simulink model "Consensus_ARdrone"  (R2017b)
settings: Solver=VariableStepAuto  StartTime=0.0  StopTime=100  MinStep=0.001  RelTol=1e-3
values from neighbouring files (symbols this model uses):
  A = zeros(n,n)    [Initial.m]    (also in matlab_promjena_form.mat = [0 1 1 1 1 1 0 1 1 1 1 1 ... (25 elements, 5x5)])
  c_d = 2.5    [Initial.m]    (also in ardrone_params.m; matlab_promjena_form.mat)
  G = zeros(n,n)    [Initial.m]    (also in matlab_promjena_form.mat = [0 0.05 0.05 0.05 0.05 0.05 0 0.05 0.05 0.05 0.05 0.05 ... ()
  g = 9.81    [Initial.m]    (also in ardrone_params.m; matlab_promjena_form.mat)
  Krug = [6.12323399574e-16 0 0 0 0 0 0 5.61829545926e-10 1.42391980871e-11 2.79677204721e-07 7.08910845246e-09 0.000111130804722 ... (72051 elements, 7x10293)]    [Krug.mat]
  m = 1.65    [Initial.m]    (also in ardrone_params.m; matlab_promjena_form.mat)
  pitch_max = 0.4    [Initial.m]    (also in ardrone_params.m; matlab_promjena_form.mat)
  R1 = [0, -1, -1, -2, -2; 0, 1,-1, 2, -2]    [Initial.m]    (also in matlab_promjena_form.mat = [0  -1  -1  -2  -2; 0  1  -1  2  -2])
  R2 = [9, 7, 5 ,3, 1; 0,0,0,0,0]    [Initial.m]    (also in matlab_promjena_form.mat = [9  7  5  3  1; 0  0  0  0  0])
  roll_max = 0.4    [Initial.m]    (also in ardrone_params.m; matlab_promjena_form.mat)
  T_pitch = 0.4    [Initial.m]    (also in ardrone_params.m; matlab_promjena_form.mat)
  T_roll = 0.4    [Initial.m]    (also in ardrone_params.m; matlab_promjena_form.mat)
  T_yaw = 0.8    [Initial.m]    (also in ardrone_params.m; matlab_promjena_form.mat)
  T_z = 0.6    [Initial.m]    (also in ardrone_params.m; matlab_promjena_form.mat)
  x0 = [20, -10, -20, 10, -20]    [Initial.m]    (also in matlab_promjena_form.mat = [0 -1 -1 -2 -2])
  y0 = [20, 10,0, -10, -20]    [Initial.m]    (also in matlab_promjena_form.mat = [0 1 -1 2 -2])
  yaw_rate_max = 0.7864    [Initial.m]    (also in ardrone_params.m; matlab_promjena_form.mat)
  z_rate_max = 0.7    [Initial.m]    (also in ardrone_params.m; matlab_promjena_form.mat)
settings Model: Creator=Mare  LastModifiedBy=Mare

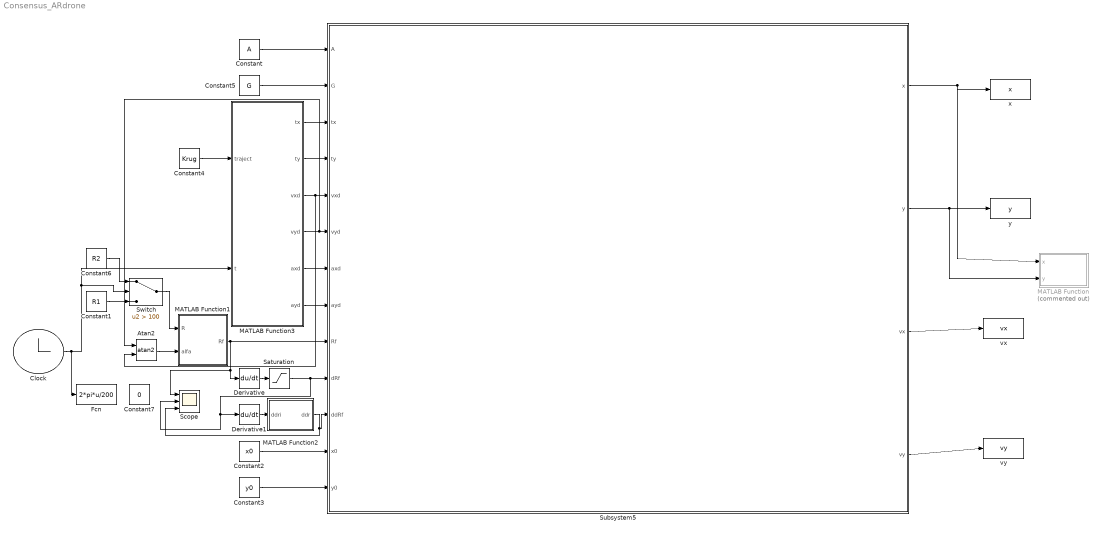
== system Consensus_ARdrone ==
  Atan2 : Trigonometry  Operator=atan2
  Clock : Clock
  Constant : Constant  Value=A
  Constant1 : Constant  Value=R1
  Constant2 : Constant  Value=x0
  Constant3 : Constant  Value=y0
  Constant4 : Constant  Value=Krug
  Constant5 : Constant  Value=G
  Constant6 : Constant  Value=R2
  Constant7 : Constant  Value=0
  Derivative : Derivative
  Derivative1 : Derivative
  Fcn : Fcn  Expr=2*pi*u/200
  MATLAB Function : MATLAB Function  Commented=on  TreatAsAtomicUnit=on
  MATLAB Function1 : MATLAB Function  TreatAsAtomicUnit=on
  MATLAB Function2 : MATLAB Function  TreatAsAtomicUnit=on
  MATLAB Function3 : MATLAB Function  TreatAsAtomicUnit=on
  Saturation : Saturate  UpperLimit=2.5  LowerLimit=-2.5
  Scope : Scope  NumInputPorts=3
  Subsystem5 : Subsystem
  Switch : Switch  Criteria=u2 > Threshold  Threshold=100
  vx : ToWorkspace  VariableName=vx  SaveFormat=Structure With Time  SampleTime=0.5
  vy : ToWorkspace  VariableName=vy  SaveFormat=Structure With Time  SampleTime=0.5
  x : ToWorkspace  VariableName=x  SaveFormat=Structure With Time  SampleTime=0.5
  y : ToWorkspace  VariableName=y  SaveFormat=Structure With Time  SampleTime=0.5
  wires:
  Constant/1 -> Subsystem5/1(A)
  MATLAB Function1/1(Rf) -> Subsystem5/9(Rf), Scope/1, Derivative/1
  Constant1/1 -> Switch/3
  Clock/1 -> Fcn/1, Switch/2, MATLAB Function3/2(t)
  Derivative/1 -> Saturation/1
  Saturation/1 -> Subsystem5/10(dRf), Scope/2, Derivative1/1
  Derivative1/1 -> MATLAB Function2/1(ddri)
  Constant3/1 -> Subsystem5/13(y0)
  Constant2/1 -> Subsystem5/12(x0)
  MATLAB Function3/6(ayd) -> Subsystem5/8(ayd)
  MATLAB Function3/5(axd) -> Subsystem5/7(axd)
  MATLAB Function3/4(vyd) -> Atan2/1, Subsystem5/6(vyd)
  MATLAB Function3/3(vxd) -> Atan2/2, Subsystem5/5(vxd)
  MATLAB Function3/2(ty) -> Subsystem5/4(ty)
  MATLAB Function3/1(tx) -> Subsystem5/3(tx)
  Constant4/1 -> MATLAB Function3/1(traject)
  Subsystem5/2(y) -> MATLAB Function/2(y), y/1
  Subsystem5/4(vy) -> vy/1
  Subsystem5/1(x) -> MATLAB Function/1(x), x/1
  Subsystem5/3(vx) -> vx/1
  Constant5/1 -> Subsystem5/2(G)
  MATLAB Function2/1(ddr) -> Subsystem5/11(ddRf), Scope/3
  Constant6/1 -> Switch/1
  Switch/1 -> MATLAB Function1/1(R)
  Atan2/1 -> MATLAB Function1/2(alfa)

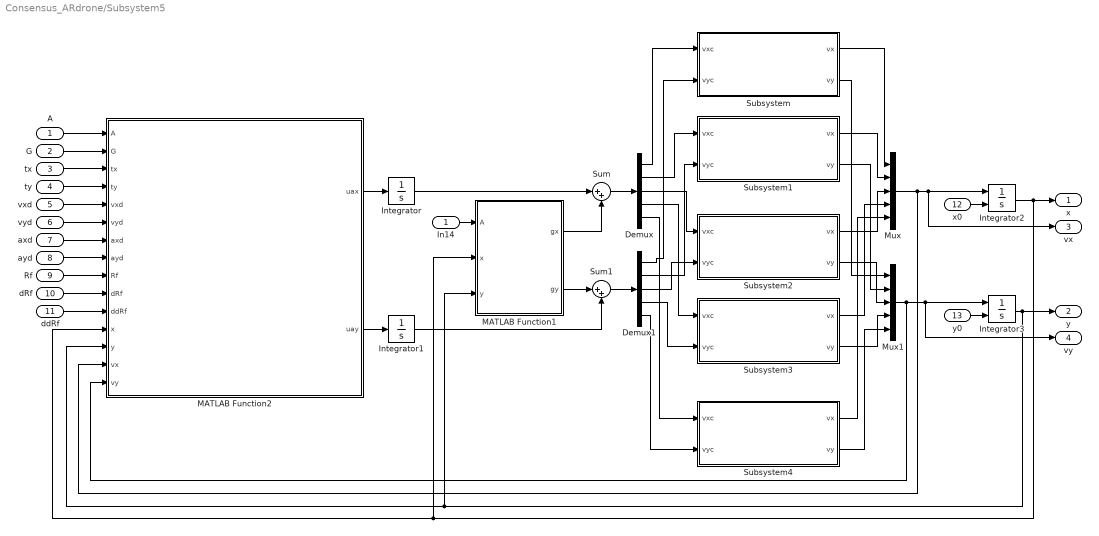
== system Consensus_ARdrone/Subsystem5 ==
  A : Inport
  G : Inport  Port=2
  tx : Inport  Port=3
  ty : Inport  Port=4
  vxd : Inport  Port=5
  vyd : Inport  Port=6
  axd : Inport  Port=7
  ayd : Inport  Port=8
  Rf : Inport  Port=9
  dRf : Inport  Port=10
  ddRf : Inport  Port=11
  x0 : Inport  Port=12
  y0 : Inport  Port=13
  Demux : Demux  Outputs=5
  Demux1 : Demux  Outputs=5
  In14 : InportShadow
  Integrator : Integrator
  Integrator1 : Integrator
  Integrator2 : Integrator  InitialConditionSource=external
  Integrator3 : Integrator  InitialConditionSource=external
  MATLAB Function1 : MATLAB Function  TreatAsAtomicUnit=on
  MATLAB Function2 : MATLAB Function  TreatAsAtomicUnit=on
  Mux : Mux  Inputs=5
  Mux1 : Mux  Inputs=5
  Subsystem : Subsystem
      mask Display: text(50, 35,'AR Drone - a1')
  Subsystem1 : Subsystem
      mask Display: text(50, 35,'AR Drone  - a2')
  Subsystem2 : Subsystem
      mask Display: text(50, 35,'AR Drone - a3')
  Subsystem3 : Subsystem
      mask Display: text(50, 35,'AR Drone  - a4')
  Subsystem4 : Subsystem
      mask Display: text(50, 35,'AR Drone - a5')
  Sum : Sum  Inputs=|++
  Sum1 : Sum  Inputs=|++
  x : Outport
  y : Outport  Port=2
  vx : Outport  Port=3
  vy : Outport  Port=4
  wires:
  Subsystem3/1("vx ") -> Mux/4
  y0/1 -> Integrator3/2
  In14/1 -> MATLAB Function1/1(A)
  vxd/1 -> MATLAB Function2/5(vxd)
  ty/1 -> MATLAB Function2/4(ty)
  Integrator2/1 -> MATLAB Function2/12(x), MATLAB Function1/2(x), x/1
  x0/1 -> Integrator2/2
  Subsystem1/2(vy) -> Mux1/2
  Subsystem3/2(vy) -> Mux1/4
  Subsystem4/2(vy) -> Mux1/5
  Subsystem2/2(vy) -> Mux1/3
  Subsystem4/1("vx ") -> Mux/5
  tx/1 -> MATLAB Function2/3(tx)
  MATLAB Function2/2(uay) -> Integrator1/1
  MATLAB Function2/1(uax) -> Integrator/1
  Subsystem2/1("vx ") -> Mux/3
  Subsystem1/1("vx ") -> Mux/2
  Rf/1 -> MATLAB Function2/9(Rf)
  dRf/1 -> MATLAB Function2/10(dRf)
  Demux1/4 -> Subsystem3/2("vyc ")
  Demux/2 -> Subsystem1/1(vxc)
  ayd/1 -> MATLAB Function2/8(ayd)
  Subsystem/1("vx ") -> Mux/1
  ddRf/1 -> MATLAB Function2/11(ddRf)
  Demux/3 -> Subsystem2/1(vxc)
  Demux/1 -> Subsystem/1(vxc)
  Mux1/1 -> vy/1, Integrator3/1, MATLAB Function2/15(vy)
  Demux/5 -> Subsystem4/1(vxc)
  Demux1/3 -> Subsystem2/2("vyc ")
  vyd/1 -> MATLAB Function2/6(vyd)
  Sum1/1 -> Demux1/1
  Subsystem/2(vy) -> Mux1/1
  Sum/1 -> Demux/1
  Integrator/1 -> Sum/1
  G/1 -> MATLAB Function2/2(G)
  MATLAB Function1/2(gy) -> Sum1/1
  Demux1/5 -> Subsystem4/2("vyc ")
  Demux/4 -> Subsystem3/1(vxc)
  axd/1 -> MATLAB Function2/7(axd)
  MATLAB Function1/1(gx) -> Sum/2
  A/1 -> MATLAB Function2/1(A)
  Demux1/1 -> Subsystem/2("vyc ")
  Integrator1/1 -> Sum1/2
  Demux1/2 -> Subsystem1/2("vyc ")
  Integrator3/1 -> y/1, MATLAB Function2/13(y), MATLAB Function1/3(y)
  Mux/1 -> vx/1, Integrator2/1, MATLAB Function2/14(vx)

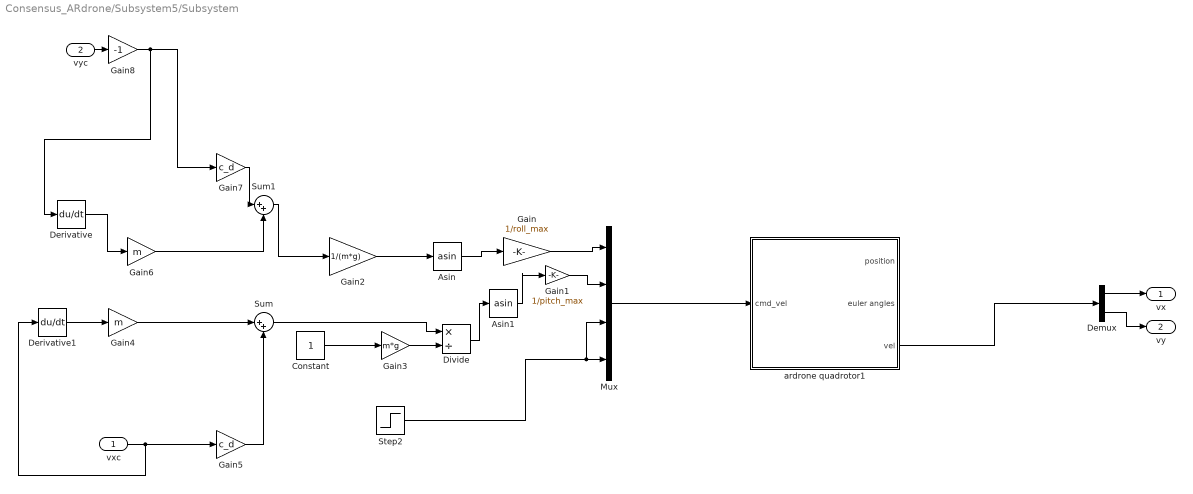
== system Consensus_ARdrone/Subsystem5/Subsystem ==
  vxc : Inport
  "vyc " : Inport  Port=2
  Asin : Trigonometry  Operator=asin
  Asin1 : Trigonometry  Operator=asin
  Constant : Constant
  Demux : Demux  Outputs=2
  Derivative : Derivative
  Derivative1 : Derivative
  Divide : Product  Inputs=*/
  Gain : Gain  Gain=1/roll_max
  Gain1 : Gain  Gain=1/pitch_max
  Gain2 : Gain  Gain=1/(m*g)
  Gain3 : Gain  Gain=m*g
  Gain4 : Gain  Gain=m
  Gain5 : Gain  Gain=c_d
  Gain6 : Gain  Gain=m
  Gain7 : Gain  Gain=c_d
  Gain8 : Gain  Gain=-1
  Mux : Mux
  Step2 : Step  Time=0  After=0  SampleTime=0
  Sum : Sum  Inputs=|++
  Sum1 : Sum  Inputs=|++
  ardrone quadrotor1 : Subsystem
  "vx " : Outport
  vy : Outport  Port=2
  wires:
  Divide/1 -> Asin1/1
  Derivative1/1 -> Gain4/1
  Gain4/1 -> Sum/1
  Constant/1 -> Gain3/1
  Gain5/1 -> Sum/2
  Mux/1 -> ardrone quadrotor1/1(cmd_vel)
  Asin/1 -> Gain/1
  Step2/1 -> Mux/3, Mux/4
  Sum1/1 -> Gain2/1
  Gain2/1 -> Asin/1
  Derivative/1 -> Gain6/1
  Gain6/1 -> Sum1/2
  Gain3/1 -> Divide/2
  vxc/1 -> Derivative1/1, Gain5/1
  Gain7/1 -> Sum1/1
  Asin1/1 -> Gain1/1
  Sum/1 -> Divide/1
  ardrone quadrotor1/3(vel) -> Demux/1
  Gain/1 -> Mux/1
  Gain1/1 -> Mux/2
  Demux/1 -> "vx "/1
  Demux/2 -> vy/1
  "vyc "/1 -> Gain8/1
  Gain8/1 -> Derivative/1, Gain7/1

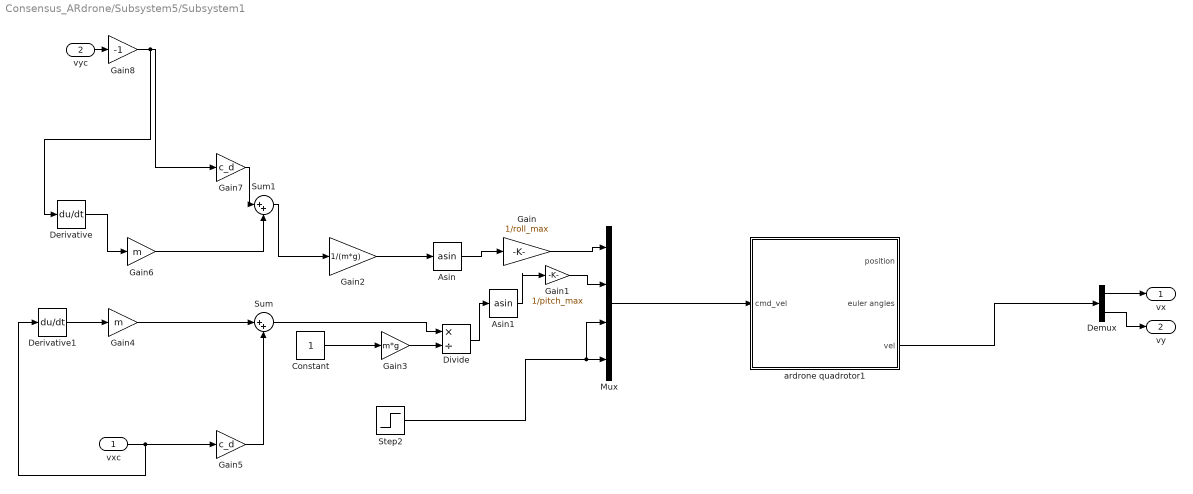
== system Consensus_ARdrone/Subsystem5/Subsystem1 ==
  vxc : Inport
  "vyc " : Inport  Port=2
  Asin : Trigonometry  Operator=asin
  Asin1 : Trigonometry  Operator=asin
  Constant : Constant
  Demux : Demux  Outputs=2
  Derivative : Derivative
  Derivative1 : Derivative
  Divide : Product  Inputs=*/
  Gain : Gain  Gain=1/roll_max
  Gain1 : Gain  Gain=1/pitch_max
  Gain2 : Gain  Gain=1/(m*g)
  Gain3 : Gain  Gain=m*g
  Gain4 : Gain  Gain=m
  Gain5 : Gain  Gain=c_d
  Gain6 : Gain  Gain=m
  Gain7 : Gain  Gain=c_d
  Gain8 : Gain  Gain=-1
  Mux : Mux
  Step2 : Step  Time=0  After=0  SampleTime=0
  Sum : Sum  Inputs=|++
  Sum1 : Sum  Inputs=|++
  ardrone quadrotor1 : Subsystem
  "vx " : Outport
  vy : Outport  Port=2
  wires:
  Divide/1 -> Asin1/1
  Derivative1/1 -> Gain4/1
  Gain4/1 -> Sum/1
  Constant/1 -> Gain3/1
  Gain5/1 -> Sum/2
  Mux/1 -> ardrone quadrotor1/1(cmd_vel)
  Asin/1 -> Gain/1
  Step2/1 -> Mux/3, Mux/4
  Sum1/1 -> Gain2/1
  Gain2/1 -> Asin/1
  Derivative/1 -> Gain6/1
  Gain6/1 -> Sum1/2
  Gain3/1 -> Divide/2
  Gain8/1 -> Derivative/1, Gain7/1
  vxc/1 -> Derivative1/1, Gain5/1
  Gain7/1 -> Sum1/1
  Asin1/1 -> Gain1/1
  Sum/1 -> Divide/1
  ardrone quadrotor1/3(vel) -> Demux/1
  Gain/1 -> Mux/1
  Gain1/1 -> Mux/2
  Demux/1 -> "vx "/1
  Demux/2 -> vy/1
  "vyc "/1 -> Gain8/1

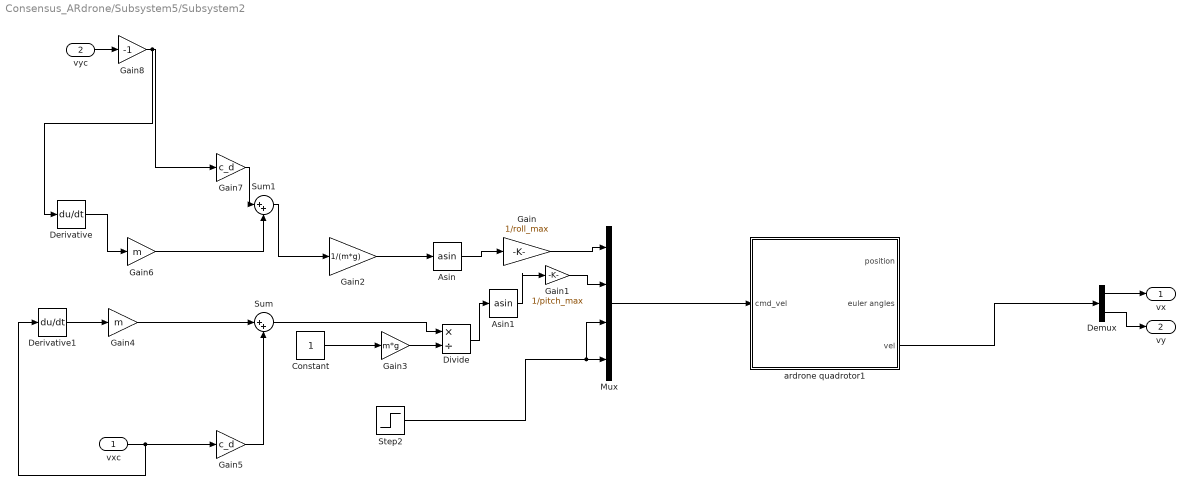
== system Consensus_ARdrone/Subsystem5/Subsystem2 ==
  vxc : Inport
  "vyc " : Inport  Port=2
  Asin : Trigonometry  Operator=asin
  Asin1 : Trigonometry  Operator=asin
  Constant : Constant
  Demux : Demux  Outputs=2
  Derivative : Derivative
  Derivative1 : Derivative
  Divide : Product  Inputs=*/
  Gain : Gain  Gain=1/roll_max
  Gain1 : Gain  Gain=1/pitch_max
  Gain2 : Gain  Gain=1/(m*g)
  Gain3 : Gain  Gain=m*g
  Gain4 : Gain  Gain=m
  Gain5 : Gain  Gain=c_d
  Gain6 : Gain  Gain=m
  Gain7 : Gain  Gain=c_d
  Gain8 : Gain  Gain=-1
  Mux : Mux
  Step2 : Step  Time=0  After=0  SampleTime=0
  Sum : Sum  Inputs=|++
  Sum1 : Sum  Inputs=|++
  ardrone quadrotor1 : Subsystem
  "vx " : Outport
  vy : Outport  Port=2
  wires:
  Divide/1 -> Asin1/1
  Derivative1/1 -> Gain4/1
  Gain4/1 -> Sum/1
  Constant/1 -> Gain3/1
  Gain5/1 -> Sum/2
  Mux/1 -> ardrone quadrotor1/1(cmd_vel)
  Asin/1 -> Gain/1
  Step2/1 -> Mux/3, Mux/4
  Sum1/1 -> Gain2/1
  Gain2/1 -> Asin/1
  Derivative/1 -> Gain6/1
  Gain6/1 -> Sum1/2
  Gain3/1 -> Divide/2
  "vyc "/1 -> Gain8/1
  vxc/1 -> Derivative1/1, Gain5/1
  Gain7/1 -> Sum1/1
  Asin1/1 -> Gain1/1
  Sum/1 -> Divide/1
  ardrone quadrotor1/3(vel) -> Demux/1
  Gain/1 -> Mux/1
  Gain1/1 -> Mux/2
  Demux/1 -> "vx "/1
  Demux/2 -> vy/1
  Gain8/1 -> Derivative/1, Gain7/1

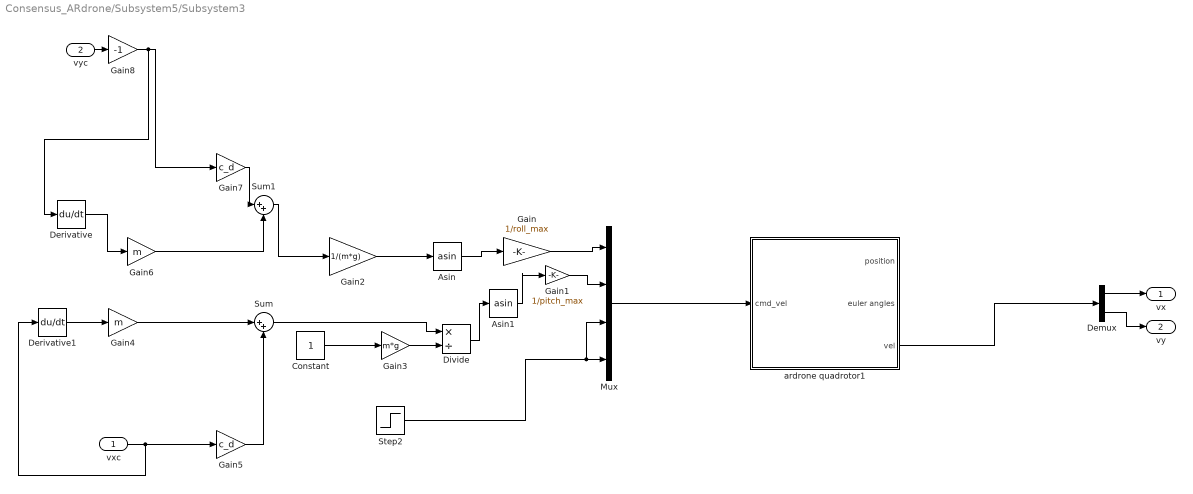
== system Consensus_ARdrone/Subsystem5/Subsystem3 ==
  vxc : Inport
  "vyc " : Inport  Port=2
  Asin : Trigonometry  Operator=asin
  Asin1 : Trigonometry  Operator=asin
  Constant : Constant
  Demux : Demux  Outputs=2
  Derivative : Derivative
  Derivative1 : Derivative
  Divide : Product  Inputs=*/
  Gain : Gain  Gain=1/roll_max
  Gain1 : Gain  Gain=1/pitch_max
  Gain2 : Gain  Gain=1/(m*g)
  Gain3 : Gain  Gain=m*g
  Gain4 : Gain  Gain=m
  Gain5 : Gain  Gain=c_d
  Gain6 : Gain  Gain=m
  Gain7 : Gain  Gain=c_d
  Gain8 : Gain  Gain=-1
  Mux : Mux
  Step2 : Step  Time=0  After=0  SampleTime=0
  Sum : Sum  Inputs=|++
  Sum1 : Sum  Inputs=|++
  ardrone quadrotor1 : Subsystem
  "vx " : Outport
  vy : Outport  Port=2
  wires:
  Divide/1 -> Asin1/1
  Derivative1/1 -> Gain4/1
  Gain4/1 -> Sum/1
  Constant/1 -> Gain3/1
  Gain5/1 -> Sum/2
  Mux/1 -> ardrone quadrotor1/1(cmd_vel)
  Asin/1 -> Gain/1
  Step2/1 -> Mux/3, Mux/4
  Sum1/1 -> Gain2/1
  Gain2/1 -> Asin/1
  Derivative/1 -> Gain6/1
  Gain6/1 -> Sum1/2
  Gain3/1 -> Divide/2
  Gain8/1 -> Derivative/1, Gain7/1
  vxc/1 -> Derivative1/1, Gain5/1
  Gain7/1 -> Sum1/1
  Asin1/1 -> Gain1/1
  Sum/1 -> Divide/1
  ardrone quadrotor1/3(vel) -> Demux/1
  Gain/1 -> Mux/1
  Gain1/1 -> Mux/2
  Demux/1 -> "vx "/1
  Demux/2 -> vy/1
  "vyc "/1 -> Gain8/1

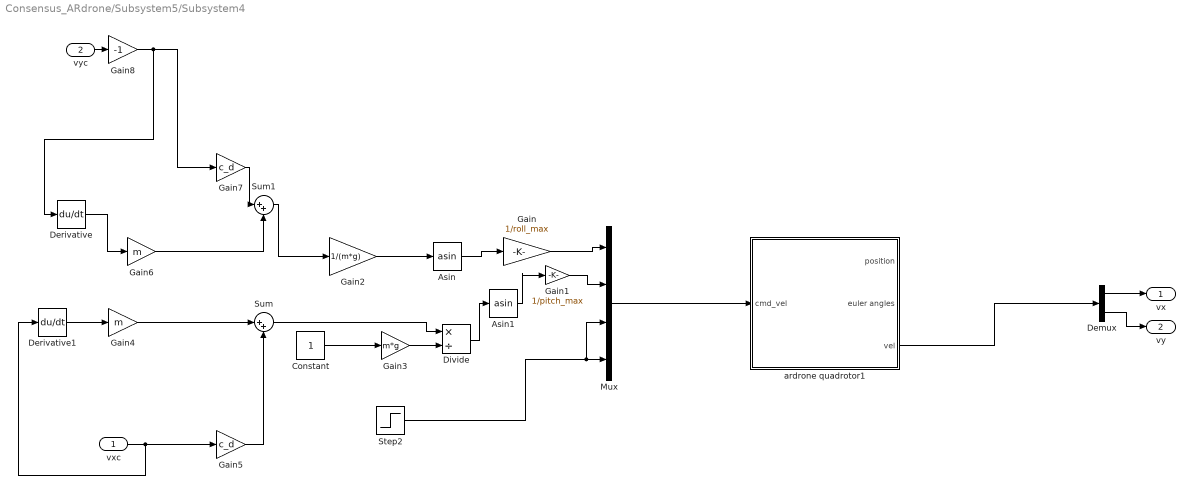
== system Consensus_ARdrone/Subsystem5/Subsystem4 ==
  vxc : Inport
  "vyc " : Inport  Port=2
  Asin : Trigonometry  Operator=asin
  Asin1 : Trigonometry  Operator=asin
  Constant : Constant
  Demux : Demux  Outputs=2
  Derivative : Derivative
  Derivative1 : Derivative
  Divide : Product  Inputs=*/
  Gain : Gain  Gain=1/roll_max
  Gain1 : Gain  Gain=1/pitch_max
  Gain2 : Gain  Gain=1/(m*g)
  Gain3 : Gain  Gain=m*g
  Gain4 : Gain  Gain=m
  Gain5 : Gain  Gain=c_d
  Gain6 : Gain  Gain=m
  Gain7 : Gain  Gain=c_d
  Gain8 : Gain  Gain=-1
  Mux : Mux
  Step2 : Step  Time=0  After=0  SampleTime=0
  Sum : Sum  Inputs=|++
  Sum1 : Sum  Inputs=|++
  ardrone quadrotor1 : Subsystem
  "vx " : Outport
  vy : Outport  Port=2
  wires:
  Divide/1 -> Asin1/1
  Derivative1/1 -> Gain4/1
  Gain4/1 -> Sum/1
  Constant/1 -> Gain3/1
  Gain5/1 -> Sum/2
  Mux/1 -> ardrone quadrotor1/1(cmd_vel)
  Asin/1 -> Gain/1
  Step2/1 -> Mux/3, Mux/4
  Sum1/1 -> Gain2/1
  Gain2/1 -> Asin/1
  Derivative/1 -> Gain6/1
  Gain6/1 -> Sum1/2
  Gain3/1 -> Divide/2
  vxc/1 -> Derivative1/1, Gain5/1
  Gain7/1 -> Sum1/1
  Asin1/1 -> Gain1/1
  Sum/1 -> Divide/1
  ardrone quadrotor1/3(vel) -> Demux/1
  Gain/1 -> Mux/1
  Gain1/1 -> Mux/2
  Demux/1 -> "vx "/1
  Demux/2 -> vy/1
  Gain8/1 -> Derivative/1, Gain7/1
  "vyc "/1 -> Gain8/1

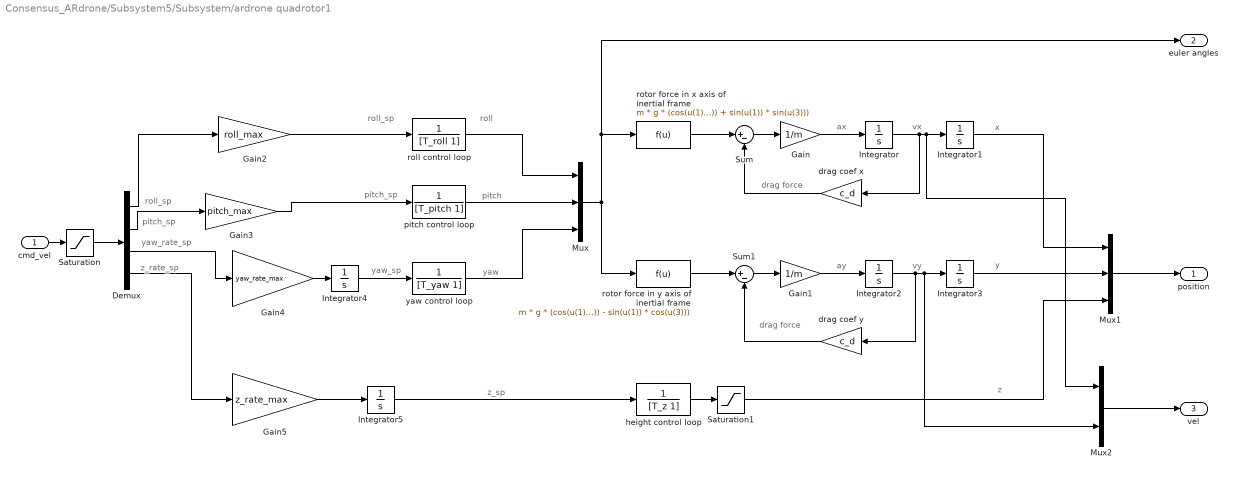
== system Consensus_ARdrone/Subsystem5/Subsystem/ardrone quadrotor1 ==
  note: pitch_sp
  note: roll_sp
  note: z_sp
  note: yaw_sp
  note: pitch_sp
  note: roll_sp
  note: z
  note: y
  note: x
  note: z_rate_sp
  note: yaw_rate_sp
  note: drag force
  note: drag force
  note: vx
  note: ax
  note: yaw
  note: pitch
  note: roll
  note: vy
  note: ay
  cmd_vel : Inport
  Demux : Demux
  Gain : Gain  Gain=1/m
  Gain1 : Gain  Gain=1/m
  Gain2 : Gain  Gain=roll_max
  Gain3 : Gain  Gain=pitch_max
  Gain4 : Gain  Gain=yaw_rate_max
  Gain5 : Gain  Gain=z_rate_max
  Integrator{,1..5} (6 alike) : Integrator
  Mux : Mux  Inputs=3
  Mux1 : Mux  Inputs=3
  Mux2 : Mux  Inputs=2
  Saturation : Saturate  UpperLimit=1  LowerLimit=-1
  Saturation1 : Saturate  UpperLimit=Inf  LowerLimit=0
  Sum : Sum  Inputs=|+-
  Sum1 : Sum  Inputs=|+-
  drag coef x : Gain  Gain=c_d
  drag coef y : Gain  Gain=c_d
  height control loop : TransferFcn  Denominator=[T_z 1]
  pitch control loop : TransferFcn  Denominator=[T_pitch 1]
  roll control loop : TransferFcn  Denominator=[T_roll 1]
  rotor force in x axis of inertial frame : Fcn  Expr=m * g * (cos(u(1)) * sin(u(2)) * cos (u(3)) + sin(u(1)) * sin(u(3)))
  rotor force in y axis of inertial frame : Fcn  Expr=m * g * (cos(u(1)) * sin(u(2)) * sin (u(3)) - sin(u(1)) * cos(u(3)))
  yaw control loop : TransferFcn  Denominator=[T_yaw 1]
  position : Outport
  euler angles : Outport  Port=2
  vel : Outport  Port=3
  wires:
  Gain1/1 -> Integrator2/1
  Integrator2/1 -> drag coef y/1, Mux2/2, Integrator3/1
  drag coef x/1 -> Sum/2
  Mux/1 -> rotor force in y axis of inertial frame/1, euler angles/1, rotor force in x axis of inertial frame/1
  pitch control loop/1 -> Mux/2
  yaw control loop/1 -> Mux/3
  rotor force in y axis of inertial frame/1 -> Sum1/1
  Sum/1 -> Gain/1
  roll control loop/1 -> Mux/1
  rotor force in x axis of inertial frame/1 -> Sum/1
  drag coef y/1 -> Sum1/2
  Gain/1 -> Integrator/1
  Sum1/1 -> Gain1/1
  Demux/3 -> Gain4/1
  Demux/4 -> Gain5/1
  Integrator1/1 -> Mux1/1
  Integrator3/1 -> Mux1/2
  height control loop/1 -> Saturation1/1
  Mux1/1 -> position/1
  Integrator/1 -> drag coef x/1, Mux2/1, Integrator1/1
  Demux/1 -> Gain2/1
  Demux/2 -> Gain3/1
  Integrator4/1 -> yaw control loop/1
  Gain4/1 -> Integrator4/1
  Gain5/1 -> Integrator5/1
  Integrator5/1 -> height control loop/1
  cmd_vel/1 -> Saturation/1
  Saturation1/1 -> Mux1/3
  Mux2/1 -> vel/1
  Saturation/1 -> Demux/1
  Gain2/1 -> roll control loop/1
  Gain3/1 -> pitch control loop/1

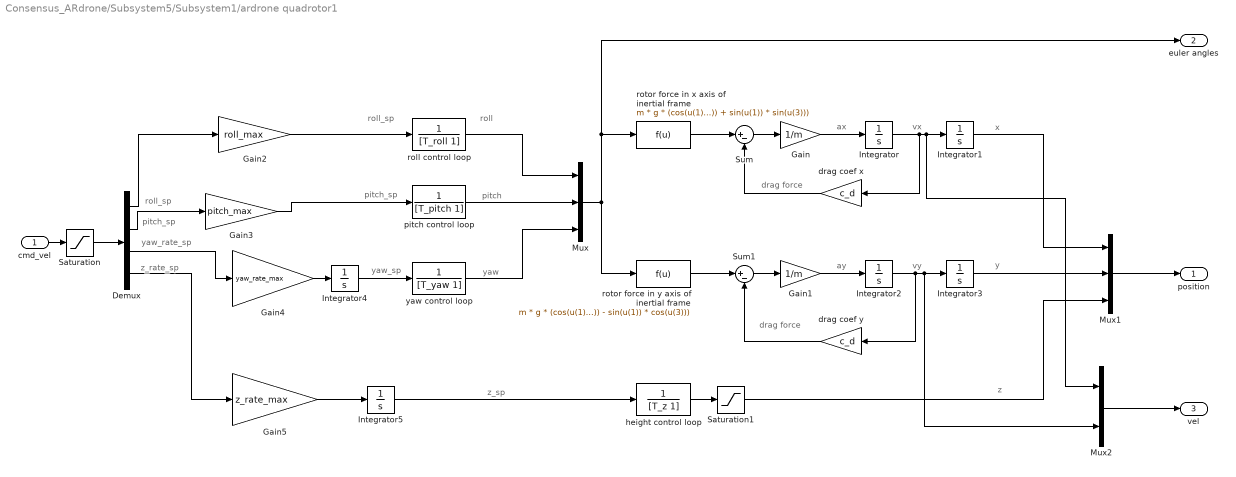
== system Consensus_ARdrone/Subsystem5/Subsystem1/ardrone quadrotor1 ==
  note: pitch_sp
  note: roll_sp
  note: z_sp
  note: yaw_sp
  note: pitch_sp
  note: roll_sp
  note: z
  note: y
  note: x
  note: z_rate_sp
  note: yaw_rate_sp
  note: drag force
  note: drag force
  note: vx
  note: ax
  note: yaw
  note: pitch
  note: roll
  note: vy
  note: ay
  cmd_vel : Inport
  Demux : Demux
  Gain : Gain  Gain=1/m
  Gain1 : Gain  Gain=1/m
  Gain2 : Gain  Gain=roll_max
  Gain3 : Gain  Gain=pitch_max
  Gain4 : Gain  Gain=yaw_rate_max
  Gain5 : Gain  Gain=z_rate_max
  Integrator{,1..5} (6 alike) : Integrator
  Mux : Mux  Inputs=3
  Mux1 : Mux  Inputs=3
  Mux2 : Mux  Inputs=2
  Saturation : Saturate  UpperLimit=1  LowerLimit=-1
  Saturation1 : Saturate  UpperLimit=Inf  LowerLimit=0
  Sum : Sum  Inputs=|+-
  Sum1 : Sum  Inputs=|+-
  drag coef x : Gain  Gain=c_d
  drag coef y : Gain  Gain=c_d
  height control loop : TransferFcn  Denominator=[T_z 1]
  pitch control loop : TransferFcn  Denominator=[T_pitch 1]
  roll control loop : TransferFcn  Denominator=[T_roll 1]
  rotor force in x axis of inertial frame : Fcn  Expr=m * g * (cos(u(1)) * sin(u(2)) * cos (u(3)) + sin(u(1)) * sin(u(3)))
  rotor force in y axis of inertial frame : Fcn  Expr=m * g * (cos(u(1)) * sin(u(2)) * sin (u(3)) - sin(u(1)) * cos(u(3)))
  yaw control loop : TransferFcn  Denominator=[T_yaw 1]
  position : Outport
  euler angles : Outport  Port=2
  vel : Outport  Port=3
  wires:
  Gain1/1 -> Integrator2/1
  Integrator2/1 -> drag coef y/1, Mux2/2, Integrator3/1
  drag coef x/1 -> Sum/2
  Mux/1 -> rotor force in y axis of inertial frame/1, euler angles/1, rotor force in x axis of inertial frame/1
  pitch control loop/1 -> Mux/2
  yaw control loop/1 -> Mux/3
  rotor force in y axis of inertial frame/1 -> Sum1/1
  Sum/1 -> Gain/1
  roll control loop/1 -> Mux/1
  rotor force in x axis of inertial frame/1 -> Sum/1
  drag coef y/1 -> Sum1/2
  Gain/1 -> Integrator/1
  Sum1/1 -> Gain1/1
  Demux/3 -> Gain4/1
  Demux/4 -> Gain5/1
  Integrator1/1 -> Mux1/1
  Integrator3/1 -> Mux1/2
  height control loop/1 -> Saturation1/1
  Mux1/1 -> position/1
  Integrator/1 -> drag coef x/1, Mux2/1, Integrator1/1
  Demux/1 -> Gain2/1
  Demux/2 -> Gain3/1
  Integrator4/1 -> yaw control loop/1
  Gain4/1 -> Integrator4/1
  Gain5/1 -> Integrator5/1
  Integrator5/1 -> height control loop/1
  cmd_vel/1 -> Saturation/1
  Saturation1/1 -> Mux1/3
  Mux2/1 -> vel/1
  Saturation/1 -> Demux/1
  Gain2/1 -> roll control loop/1
  Gain3/1 -> pitch control loop/1

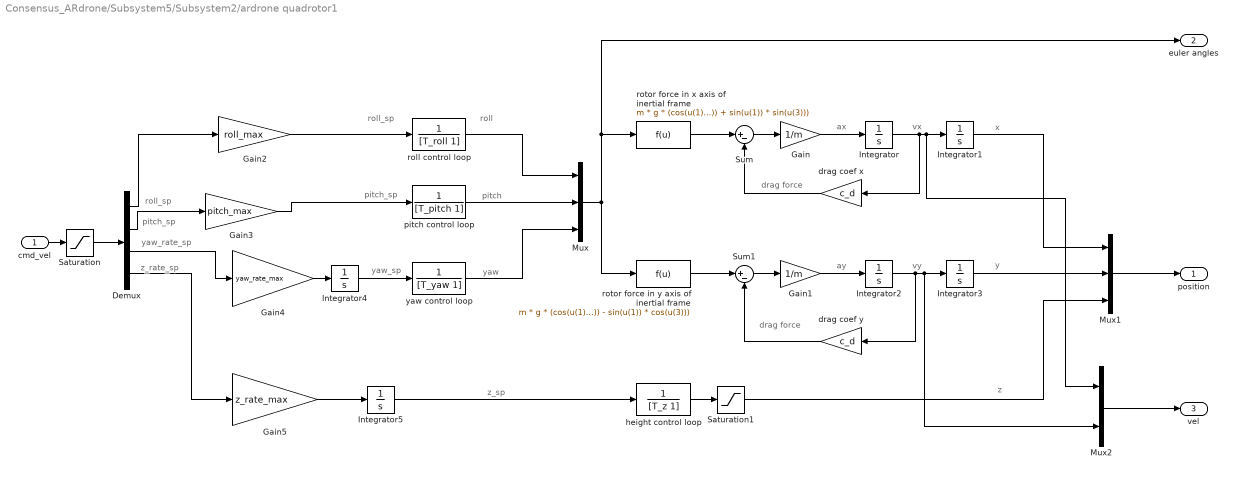
== system Consensus_ARdrone/Subsystem5/Subsystem2/ardrone quadrotor1 ==
  note: pitch_sp
  note: roll_sp
  note: z_sp
  note: yaw_sp
  note: pitch_sp
  note: roll_sp
  note: z
  note: y
  note: x
  note: z_rate_sp
  note: yaw_rate_sp
  note: drag force
  note: drag force
  note: vx
  note: ax
  note: yaw
  note: pitch
  note: roll
  note: vy
  note: ay
  cmd_vel : Inport
  Demux : Demux
  Gain : Gain  Gain=1/m
  Gain1 : Gain  Gain=1/m
  Gain2 : Gain  Gain=roll_max
  Gain3 : Gain  Gain=pitch_max
  Gain4 : Gain  Gain=yaw_rate_max
  Gain5 : Gain  Gain=z_rate_max
  Integrator{,1..5} (6 alike) : Integrator
  Mux : Mux  Inputs=3
  Mux1 : Mux  Inputs=3
  Mux2 : Mux  Inputs=2
  Saturation : Saturate  UpperLimit=1  LowerLimit=-1
  Saturation1 : Saturate  UpperLimit=Inf  LowerLimit=0
  Sum : Sum  Inputs=|+-
  Sum1 : Sum  Inputs=|+-
  drag coef x : Gain  Gain=c_d
  drag coef y : Gain  Gain=c_d
  height control loop : TransferFcn  Denominator=[T_z 1]
  pitch control loop : TransferFcn  Denominator=[T_pitch 1]
  roll control loop : TransferFcn  Denominator=[T_roll 1]
  rotor force in x axis of inertial frame : Fcn  Expr=m * g * (cos(u(1)) * sin(u(2)) * cos (u(3)) + sin(u(1)) * sin(u(3)))
  rotor force in y axis of inertial frame : Fcn  Expr=m * g * (cos(u(1)) * sin(u(2)) * sin (u(3)) - sin(u(1)) * cos(u(3)))
  yaw control loop : TransferFcn  Denominator=[T_yaw 1]
  position : Outport
  euler angles : Outport  Port=2
  vel : Outport  Port=3
  wires:
  Gain1/1 -> Integrator2/1
  Integrator2/1 -> drag coef y/1, Mux2/2, Integrator3/1
  drag coef x/1 -> Sum/2
  Mux/1 -> rotor force in y axis of inertial frame/1, euler angles/1, rotor force in x axis of inertial frame/1
  pitch control loop/1 -> Mux/2
  yaw control loop/1 -> Mux/3
  rotor force in y axis of inertial frame/1 -> Sum1/1
  Sum/1 -> Gain/1
  roll control loop/1 -> Mux/1
  rotor force in x axis of inertial frame/1 -> Sum/1
  drag coef y/1 -> Sum1/2
  Gain/1 -> Integrator/1
  Sum1/1 -> Gain1/1
  Demux/3 -> Gain4/1
  Demux/4 -> Gain5/1
  Integrator1/1 -> Mux1/1
  Integrator3/1 -> Mux1/2
  height control loop/1 -> Saturation1/1
  Mux1/1 -> position/1
  Integrator/1 -> drag coef x/1, Mux2/1, Integrator1/1
  Demux/1 -> Gain2/1
  Demux/2 -> Gain3/1
  Integrator4/1 -> yaw control loop/1
  Gain4/1 -> Integrator4/1
  Gain5/1 -> Integrator5/1
  Integrator5/1 -> height control loop/1
  cmd_vel/1 -> Saturation/1
  Saturation1/1 -> Mux1/3
  Mux2/1 -> vel/1
  Saturation/1 -> Demux/1
  Gain2/1 -> roll control loop/1
  Gain3/1 -> pitch control loop/1

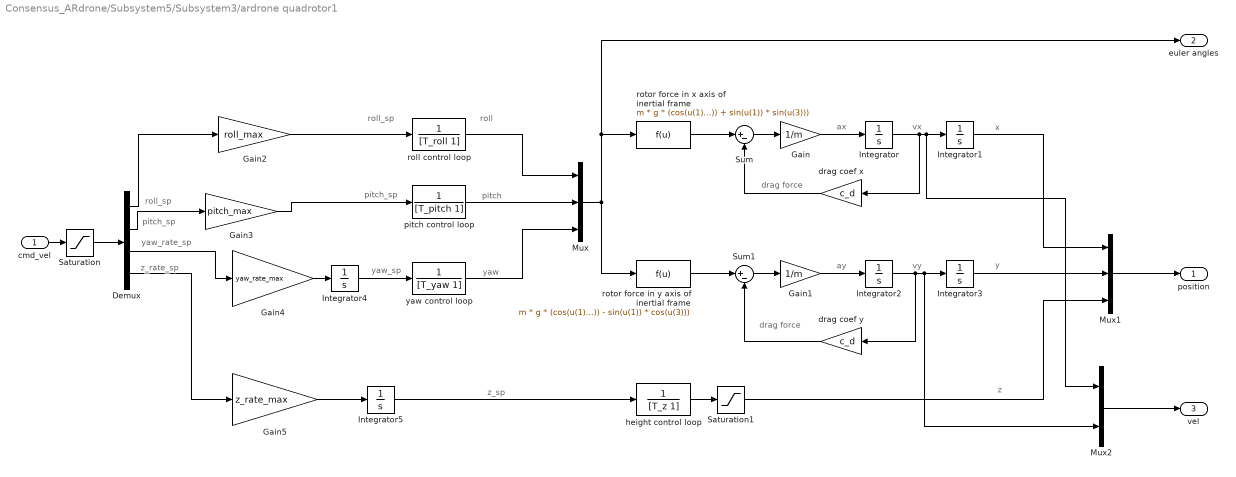
== system Consensus_ARdrone/Subsystem5/Subsystem3/ardrone quadrotor1 ==
  note: pitch_sp
  note: roll_sp
  note: z_sp
  note: yaw_sp
  note: pitch_sp
  note: roll_sp
  note: z
  note: y
  note: x
  note: z_rate_sp
  note: yaw_rate_sp
  note: drag force
  note: drag force
  note: vx
  note: ax
  note: yaw
  note: pitch
  note: roll
  note: vy
  note: ay
  cmd_vel : Inport
  Demux : Demux
  Gain : Gain  Gain=1/m
  Gain1 : Gain  Gain=1/m
  Gain2 : Gain  Gain=roll_max
  Gain3 : Gain  Gain=pitch_max
  Gain4 : Gain  Gain=yaw_rate_max
  Gain5 : Gain  Gain=z_rate_max
  Integrator{,1..5} (6 alike) : Integrator
  Mux : Mux  Inputs=3
  Mux1 : Mux  Inputs=3
  Mux2 : Mux  Inputs=2
  Saturation : Saturate  UpperLimit=1  LowerLimit=-1
  Saturation1 : Saturate  UpperLimit=Inf  LowerLimit=0
  Sum : Sum  Inputs=|+-
  Sum1 : Sum  Inputs=|+-
  drag coef x : Gain  Gain=c_d
  drag coef y : Gain  Gain=c_d
  height control loop : TransferFcn  Denominator=[T_z 1]
  pitch control loop : TransferFcn  Denominator=[T_pitch 1]
  roll control loop : TransferFcn  Denominator=[T_roll 1]
  rotor force in x axis of inertial frame : Fcn  Expr=m * g * (cos(u(1)) * sin(u(2)) * cos (u(3)) + sin(u(1)) * sin(u(3)))
  rotor force in y axis of inertial frame : Fcn  Expr=m * g * (cos(u(1)) * sin(u(2)) * sin (u(3)) - sin(u(1)) * cos(u(3)))
  yaw control loop : TransferFcn  Denominator=[T_yaw 1]
  position : Outport
  euler angles : Outport  Port=2
  vel : Outport  Port=3
  wires:
  Gain1/1 -> Integrator2/1
  Integrator2/1 -> drag coef y/1, Mux2/2, Integrator3/1
  drag coef x/1 -> Sum/2
  Mux/1 -> rotor force in y axis of inertial frame/1, euler angles/1, rotor force in x axis of inertial frame/1
  pitch control loop/1 -> Mux/2
  yaw control loop/1 -> Mux/3
  rotor force in y axis of inertial frame/1 -> Sum1/1
  Sum/1 -> Gain/1
  roll control loop/1 -> Mux/1
  rotor force in x axis of inertial frame/1 -> Sum/1
  drag coef y/1 -> Sum1/2
  Gain/1 -> Integrator/1
  Sum1/1 -> Gain1/1
  Demux/3 -> Gain4/1
  Demux/4 -> Gain5/1
  Integrator1/1 -> Mux1/1
  Integrator3/1 -> Mux1/2
  height control loop/1 -> Saturation1/1
  Mux1/1 -> position/1
  Integrator/1 -> drag coef x/1, Mux2/1, Integrator1/1
  Demux/1 -> Gain2/1
  Demux/2 -> Gain3/1
  Integrator4/1 -> yaw control loop/1
  Gain4/1 -> Integrator4/1
  Gain5/1 -> Integrator5/1
  Integrator5/1 -> height control loop/1
  cmd_vel/1 -> Saturation/1
  Saturation1/1 -> Mux1/3
  Mux2/1 -> vel/1
  Saturation/1 -> Demux/1
  Gain2/1 -> roll control loop/1
  Gain3/1 -> pitch control loop/1

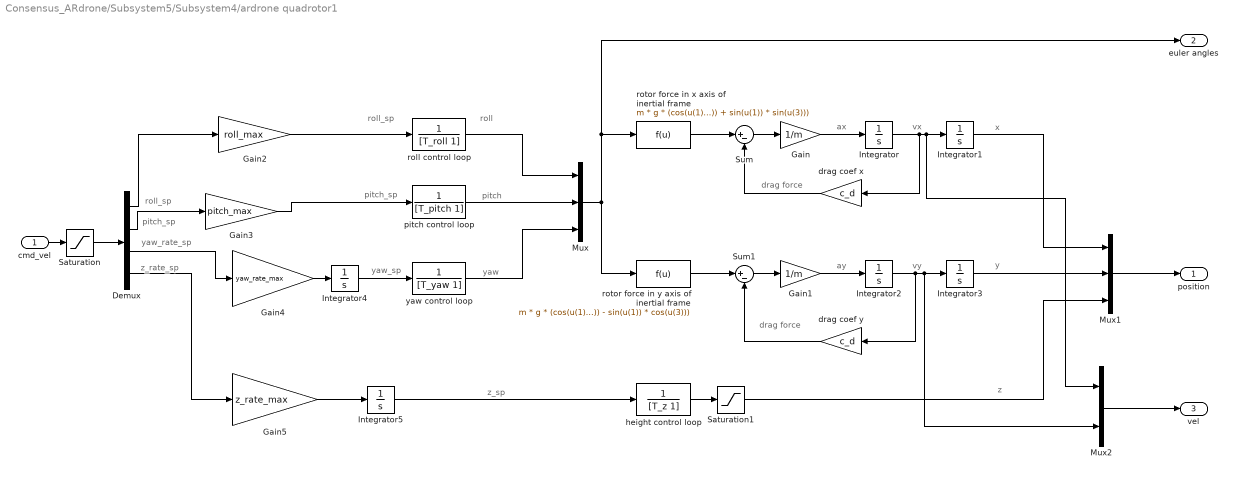
== system Consensus_ARdrone/Subsystem5/Subsystem4/ardrone quadrotor1 ==
  note: pitch_sp
  note: roll_sp
  note: z_sp
  note: yaw_sp
  note: pitch_sp
  note: roll_sp
  note: z
  note: y
  note: x
  note: z_rate_sp
  note: yaw_rate_sp
  note: drag force
  note: drag force
  note: vx
  note: ax
  note: yaw
  note: pitch
  note: roll
  note: vy
  note: ay
  cmd_vel : Inport
  Demux : Demux
  Gain : Gain  Gain=1/m
  Gain1 : Gain  Gain=1/m
  Gain2 : Gain  Gain=roll_max
  Gain3 : Gain  Gain=pitch_max
  Gain4 : Gain  Gain=yaw_rate_max
  Gain5 : Gain  Gain=z_rate_max
  Integrator{,1..5} (6 alike) : Integrator
  Mux : Mux  Inputs=3
  Mux1 : Mux  Inputs=3
  Mux2 : Mux  Inputs=2
  Saturation : Saturate  UpperLimit=1  LowerLimit=-1
  Saturation1 : Saturate  UpperLimit=Inf  LowerLimit=0
  Sum : Sum  Inputs=|+-
  Sum1 : Sum  Inputs=|+-
  drag coef x : Gain  Gain=c_d
  drag coef y : Gain  Gain=c_d
  height control loop : TransferFcn  Denominator=[T_z 1]
  pitch control loop : TransferFcn  Denominator=[T_pitch 1]
  roll control loop : TransferFcn  Denominator=[T_roll 1]
  rotor force in x axis of inertial frame : Fcn  Expr=m * g * (cos(u(1)) * sin(u(2)) * cos (u(3)) + sin(u(1)) * sin(u(3)))
  rotor force in y axis of inertial frame : Fcn  Expr=m * g * (cos(u(1)) * sin(u(2)) * sin (u(3)) - sin(u(1)) * cos(u(3)))
  yaw control loop : TransferFcn  Denominator=[T_yaw 1]
  position : Outport
  euler angles : Outport  Port=2
  vel : Outport  Port=3
  wires:
  Gain1/1 -> Integrator2/1
  Integrator2/1 -> drag coef y/1, Mux2/2, Integrator3/1
  drag coef x/1 -> Sum/2
  Mux/1 -> rotor force in y axis of inertial frame/1, euler angles/1, rotor force in x axis of inertial frame/1
  pitch control loop/1 -> Mux/2
  yaw control loop/1 -> Mux/3
  rotor force in y axis of inertial frame/1 -> Sum1/1
  Sum/1 -> Gain/1
  roll control loop/1 -> Mux/1
  rotor force in x axis of inertial frame/1 -> Sum/1
  drag coef y/1 -> Sum1/2
  Gain/1 -> Integrator/1
  Sum1/1 -> Gain1/1
  Demux/3 -> Gain4/1
  Demux/4 -> Gain5/1
  Integrator1/1 -> Mux1/1
  Integrator3/1 -> Mux1/2
  height control loop/1 -> Saturation1/1
  Mux1/1 -> position/1
  Integrator/1 -> drag coef x/1, Mux2/1, Integrator1/1
  Demux/1 -> Gain2/1
  Demux/2 -> Gain3/1
  Integrator4/1 -> yaw control loop/1
  Gain4/1 -> Integrator4/1
  Gain5/1 -> Integrator5/1
  Integrator5/1 -> height control loop/1
  cmd_vel/1 -> Saturation/1
  Saturation1/1 -> Mux1/3
  Mux2/1 -> vel/1
  Saturation/1 -> Demux/1
  Gain2/1 -> roll control loop/1
  Gain3/1 -> pitch control loop/1

== matlab function Consensus_ARdrone/MATLAB Function ==
  data: x input; y input
function  fcn(x,y)
%postavljanje granicnih vrijednosti koordinata
xmax = 25;
xmin = -25;
ymax = 25;
ymin = -10;

colors = {[0.6,0.9,0.6],[0,0.7,1],[0.85, 0.6,0.85],[1,0.8,0],[0.9,0.6,0.5], [0,1,0],[1,0,0]};


cla;
axis([xmin,xmax,ymin,ymax]);
xlabel('x');
ylabel('y');
grid on;

for k = 1:length(x)
    plot(x(k),y(k),'o', 'Color', colors{k});
    hold on;
end
% k = [0:0.1:200];
% xt = 10*cos(2*pi*k/500-pi/2);
% yt = 10*sin(2*pi*k/500-pi/2) + 10;
% plot(xt,yt)
% plot((45:1:75), 1.5, 'x');
% plot((45:1:75), -1.5, 'x');

coder.extrinsic('legend');
legend('a1', 'a2', 'a3', 'a4','a5');

== matlab function Consensus_ARdrone/Subsystem5/MATLAB Function2 ==
  data: uax output; A input; G input; tx input; ty input; vxd input; vyd input; uay output; axd input; ayd input; Rf input; dRf input; ddRf input; x input; y input; vx input; vy input
function [uax,uay]= fcn(A,G, tx,ty,vxd,vyd,axd, ayd, Rf,dRf,ddRf,x,y,vx,vy)
uax=zeros(1,length(A));
uay = zeros(1, length(A));
%azout = zeros(length(A),1);
beta = 1;
gama = 1;



for i = 1:length(A)
    uax(i) = (ddRf(1,i)+axd - beta*(x(i)-(Rf(1,i)+tx)) - gama*beta*(vx(i)-dRf(1,i)-vxd));
    uay(i) = (ddRf(2,i)+ayd - beta*(y(i)-(Rf(2,i)+ty)) - gama*beta*(vy(i)-dRf(2,i)-vyd));
    %azout(i) = 0 - C(i)*vz(i);
    for j = 1:length(A)
        uax(i) = uax(i) - 1*A(i,j)*((x(i)-Rf(1,i))-(x(j)-Rf(1,j))+ gama*((vx(i)-dRf(1,i))-(vx(j)-dRf(1,j))));
        uay(i) = uay(i) - 1*A(i,j)*((y(i)-Rf(2,i))-(y(j)-Rf(2,j))+ gama*((vy(i)-dRf(2,i))-(vy(j)-dRf(2,j))));
        %azout(i) = azout(i) - A(i,j)*(B(j)*(z(i)-R(3,i))-(y(j)-R(3,j))+ C(j)*(vz(i)-vz(j)));
    end
end

== matlab function Consensus_ARdrone/Subsystem5/MATLAB Function1 ==
  data: A input; x input; gx output; y input; gy output
function [gx, gy]= fcn(A,x,y)
%funkcija potencijala
gx = zeros(length(A),1);
gy = zeros(length(A),1);


for i = 1:length(x)
  for j = 1:length(x)
      if sqrt((x(i)-x(j))^2+(y(i)-y(j))^2)<1.2&& j ~= i
            gx(i) = gx(i) + A(i,j)*(1.2/sqrt((x(i)-x(j))^2+(y(i)-y(j))^2)-1)*1.2/sqrt((x(i)-x(j))^2+(y(i)-y(j))^2)^3*(x(i)-x(j));
            gy(i) = gy(i) + A(i,j)*(1.2/sqrt((x(i)-x(j))^2+(y(i)-y(j))^2)-1)*1.2/sqrt((x(i)-x(j))^2+(y(i)-y(j))^2)^3*(y(i)-y(j));
      end
  end
end

== matlab function Consensus_ARdrone/MATLAB Function1 ==
  data: Rf output; R input; alfa input
function Rf = fcn( R, alfa)
T = [cos(alfa), -sin(alfa);sin(alfa),cos(alfa)];
Rf = T*R;

== matlab function Consensus_ARdrone/MATLAB Function3 ==
  data: tx output; traject input; t input; ty output; vxd output; vyd output; axd output; ayd output
function [tx, ty, vxd, vyd, axd, ayd]= fcn( traject, t)
% if t<50
%     tx = 0;
%     ty = 0;
%     vxd = 0;
%     vyd = 0;
%     axd = 0;
%     ayd = 0;
% else
    tx = traject(1,ceil(t*100)+1);
    ty = traject(2,ceil(t*100)+1);
    vxd = traject(3,ceil(t*100)+1);
    vyd = traject(4,ceil(t*100)+1);
    axd = traject(5,ceil(t*100)+1);
    ayd = traject(6,ceil(t*100)+1);
% end

% tx = 0;
% ty = 0;
% vxd = 0.5;
% vyd = 0;
% axd = 0;
% ayd = 0;

== matlab function Consensus_ARdrone/MATLAB Function2 ==
  data: ddri input; ddr output
function ddr = fcn(ddri)
ddr = zeros(2,5);
for i = 1:5
    if abs(ddri(1,i))>0.2
        ddr(1,i) = 0;
    else
        ddr(1,i) = ddri(1,i);
    end
    if abs(ddri(2, i))>0.2
        ddr(2,i) = 0;
    else
        ddr(2,i) = ddri(2,i);
    end
end
